simulink model "controller"  (R2017a)
settings: Solver=FixedStepAuto  StartTime=0.0  StopTime=10.0  FixedStep=dt  RelTol=1e-3
values from neighbouring files (symbols this model uses):
  A = eye(6,6)    [main.m]
  B = zeros(6,3)    [main.m]
  C = eye(6,6)    [main.m]
  D = B    [main.m]
  F = [-1.2;.0;0]    [main.m]
  Kd = 5*eye(3)    [main.m]
  Kp = 800000*eye(3)    [main.m]
settings Model: Creator=nathaniel  LastModifiedBy=nathaniel

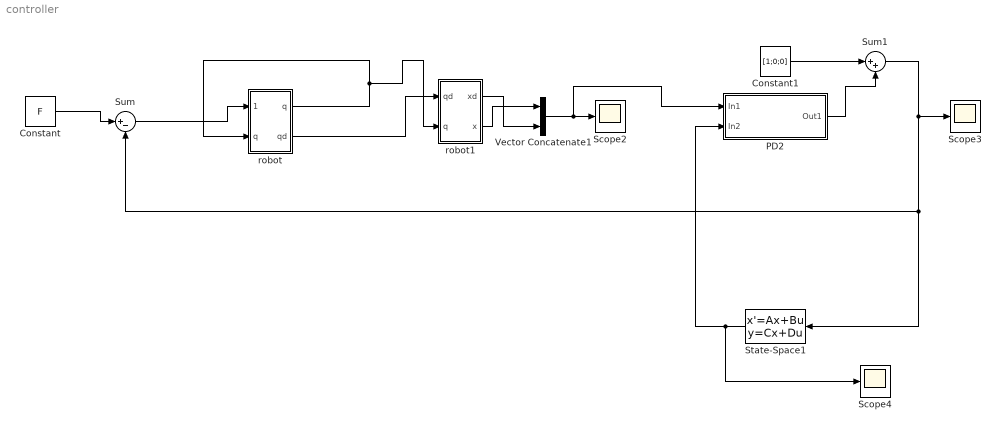
== system controller ==
  Constant : Constant  Value=F
  Constant1 : Constant  Value=[1;0;0]
  PD2 : Subsystem
  Scope2 : Scope
  Scope3 : Scope
  Scope4 : Scope
  State-Space1 : StateSpace  A=A  B=B  C=C  D=D  X0=[0;0;0;0;0;0]
  Sum : Sum  Inputs=|+-
  Sum1 : Sum  Inputs=|++
  Vector Concatenate1 : Concatenate
  robot : Subsystem
  robot1 : Subsystem
  wires:
  robot/1("q ") -> robot1/2(q), robot/2(q)
  robot/2(qd) -> robot1/1(qd)
  Constant/1 -> Sum/1
  Sum/1 -> robot/1(force)
  Vector Concatenate1/1 -> Scope2/1, PD2/1(In1)
  State-Space1/1 -> Scope4/1, PD2/2(In2)
  PD2/1(Out1) -> Sum1/2
  Sum1/1 -> Sum/2, State-Space1/1, Scope3/1
  Constant1/1 -> Sum1/1
  robot1/1(xd) -> Vector Concatenate1/2
  robot1/2(x) -> Vector Concatenate1/1

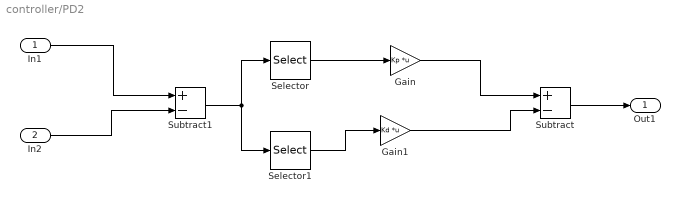
== system controller/PD2 ==
  In1 : Inport
  In2 : Inport  Port=2
  Gain : Gain  Gain=Kp  Multiplication=Matrix(K*u)
  Gain1 : Gain  Gain=Kd  Multiplication=Matrix(K*u)
  Selector : Selector  InputPortWidth=6  IndexOptions=Index vector (dialog)  Indices=[1 2 3]  OutputSizes=1
  Selector1 : Selector  InputPortWidth=6  IndexOptions=Index vector (dialog)  Indices=[4 5 6]  OutputSizes=1
  Subtract : Sum  Inputs=+-
  Subtract1 : Sum  Inputs=+-
  Out1 : Outport
  wires:
  Subtract/1 -> Out1/1
  In2/1 -> Subtract1/2
  In1/1 -> Subtract1/1
  Subtract1/1 -> Selector/1, Selector1/1
  Selector1/1 -> Gain1/1
  Selector/1 -> Gain/1
  Gain1/1 -> Subtract/2
  Gain/1 -> Subtract/1

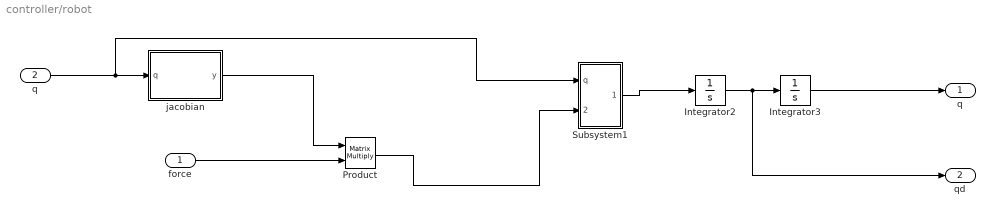
== system controller/robot ==
  force : Inport
  q : Inport  Port=2
  Integrator2 : Integrator  InitialCondition=[0;0;0]
  Integrator3 : Integrator  InitialCondition=[0;0;0]
  Product : Product  Multiplication=Matrix(*)
  Subsystem1 : Subsystem
  jacobian : MATLAB Function  TreatAsAtomicUnit=on
  "q " : Outport
  qd : Outport  Port=2
  wires:
  Subsystem1/1(qdd2) -> Integrator2/1
  Integrator2/1 -> qd/1, Integrator3/1
  Product/1 -> Subsystem1/2(tau)
  Integrator3/1 -> "q "/1
  jacobian/1(y) -> Product/1
  force/1 -> Product/2
  q/1 -> Subsystem1/1(q), jacobian/1(q)

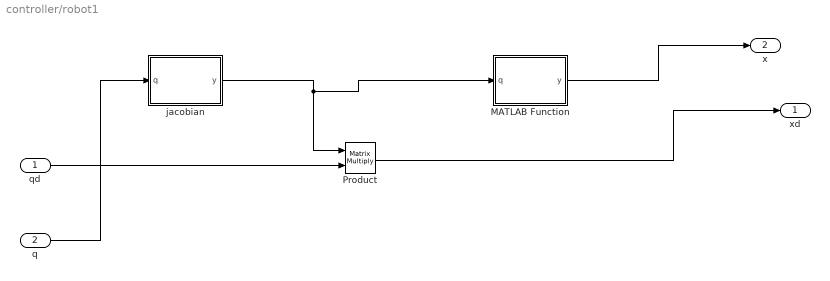
== system controller/robot1 ==
  qd : Inport
  q : Inport  Port=2
  MATLAB Function : MATLAB Function  TreatAsAtomicUnit=on
  Product : Product  Multiplication=Matrix(*)
  jacobian : MATLAB Function  TreatAsAtomicUnit=on
  xd : Outport
  x : Outport  Port=2
  wires:
  q/1 -> jacobian/1(q)
  qd/1 -> Product/2
  jacobian/1(y) -> MATLAB Function/1(q), Product/1
  Product/1 -> xd/1
  MATLAB Function/1(y) -> x/1

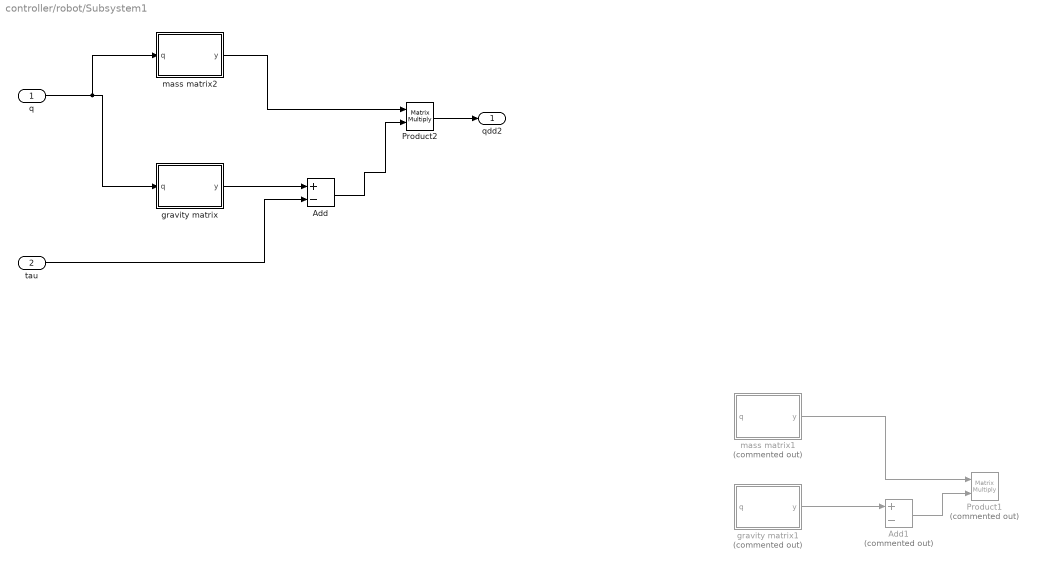
== system controller/robot/Subsystem1 ==
  q : Inport
  tau : Inport  Port=2
  Add : Sum  Inputs=+-
  Add1 : Sum  Commented=on  Inputs=+-
  Product1 : Product  Commented=on  Multiplication=Matrix(*)
  Product2 : Product  Multiplication=Matrix(*)
  gravity matrix : MATLAB Function  TreatAsAtomicUnit=on
  gravity matrix1 : MATLAB Function  Commented=on  TreatAsAtomicUnit=on
  mass matrix1 : MATLAB Function  Commented=on  TreatAsAtomicUnit=on
  mass matrix2 : MATLAB Function  TreatAsAtomicUnit=on
  qdd2 : Outport
  wires:
  gravity matrix/1(y) -> Add/1
  tau/1 -> Add/2
  Add/1 -> Product2/2
  Add1/1 -> Product1/2
  gravity matrix1/1(y) -> Add1/1
  mass matrix1/1(y) -> Product1/1
  q/1 -> mass matrix2/1(q), gravity matrix/1(q)
  mass matrix2/1(y) -> Product2/1
  Product2/1 -> qdd2/1

== matlab function controller/robot/jacobian ==
  data: q input; y output
function y = fcn(q)
  
    [j1,j2,j3] = getJ(q)  

    y = transpose(j3);

== matlab function controller/robot/Subsystem1/gravity matrix1 ==
  data: q input; y output
function y = fcn(q)
  
   
    m = 1;
    w = 2;
    h = 2.5;
    l0 = 15;
    l1 = 22;
    l2 = 17;
    l = [l0;l1;l2]; 

    g = [0;0;-9.81];
    
    [j1,j2,j3] = getJ(q)

    G1 = transpose(j1)*g;
    G2 = transpose(j2)*g;
    G3 = transpose(j3)*g;

    y = G1+G2+G3;

== matlab function controller/robot/Subsystem1/mass matrix1 ==
  data: q input; y output
function y = fcn(q)
  
   
    m = 1;
    w = 2;
    h = 2.5;
    l0 = 15;
    l1 = 22;
    l2 = 17;
    l = [l0;l1;l2]; 

    M = zeros(3,3,3);
  
    for ii = 1:3

      M(1,1,ii) = m;
      M(2,2,ii) = m;
      M(3,3,ii) = m;

    end

  
    [j1,j2,j3] = getJ(q)

    M1 = j1*M(:,:,1)*transpose(j1)
    M2 = j2*M(:,:,1)*transpose(j2)
    M3 = j3*M(:,:,1)*transpose(j3)


    y = pinv(M1+M2+M3);

== matlab function controller/robot/Subsystem1/gravity matrix ==
  data: q input; y output
function y = fcn(q)
  
   
    m = 1;
    w = 2;
    h = 2.5;
    l0 = 15;
    l1 = 22;
    l2 = 17;
    l = [l0;l1;l2]; 

    g = [0;0;-9.81];
    
    [j1,j2,j3] = getJ(q)

    G1 = transpose(j1)*g;
    G2 = transpose(j2)*g;
    G3 = transpose(j3)*g;

    y = G1+G2+G3;

== matlab function controller/robot/Subsystem1/mass matrix2 ==
  data: q input; y output
function y = fcn(q)
  
   
    m = 1;
    w = 2;
    h = 2.5;
    l0 = 15;
    l1 = 22;
    l2 = 17;
    l = [l0;l1;l2]; 

    M = zeros(3,3,3);
  
    for ii = 1:3

      M(1,1,ii) = m;
      M(2,2,ii) = m;
      M(3,3,ii) = m;

    end

  
    [j1,j2,j3] = getJ(q)

    M1 = transpose(j1)*M(:,:,1)*j1
    M2 = transpose(j2)*M(:,:,2)*transpose(j2)
    M3 = transpose(j3)*M(:,:,3)*transpose(j3)
    M = pinv(M1+M2+M3)
   

    y = M;

== matlab function controller/robot1/MATLAB Function ==
  data: q input; y output
function y = fcn(q)

y = fk(q);

== matlab function controller/robot1/jacobian ==
  data: q input; y output
function y = fcn(q)
  
    [j1,j2,j3] = getJ(q)  

    y = j3;
